simulink model "GPCA_Alarm"  (Simulink 8.5)
settings: Solver=ode45  StartTime=0.0  StopTime=10.0  RelTol=1e-3
settings Model: Creator=bourbouh  LastModifiedBy=Teme
settings DataIOCC: LimitDataPoints=off  SaveFormat=Dataset  SignalLoggingSaveFormat=Dataset
settings OptimizationCC: ExpressionDepthLimit=128
settings DebuggingCC: UnderspecifiedInitializationDetection=Simplified  MergeDetectMultiDrivingBlocksExec=error  FcnCallInpInsideContextMsg=EnableAllAsError  StateNameClashWarn=none
settings HardwareCC: ProdBitPerPointer=64  ProdLargestAtomicFloat=Float  ProdIntDivRoundTo=Zero  ProdEndianess=LittleEndian  ProdWordSize=64  ProdHWDeviceType=Intel->x86-64 (Windows64)  TargetBitPerInt=16  TargetBitPerPointer=16  TargetShiftRightIntArith=off  TargetIntDivRoundTo=Zero  TargetWordSize=8  TargetHWDeviceType=Intel->8051 Compatible  ProdEqTarget=off
settings ModelReferenceCC: PropagateSignalLabelsOutOfModel=on
settings GRTTargetCC: CombineOutputUpdateFcns=on  GRTInterface=off
settings ConfigComp: CovMetricSettings=dw  CovHtmlReporting=on  CovSaveCumulativeToWorkspaceVar=on  CovSaveSingleToWorkspaceVar=on  CovExternalEMLEnable=off

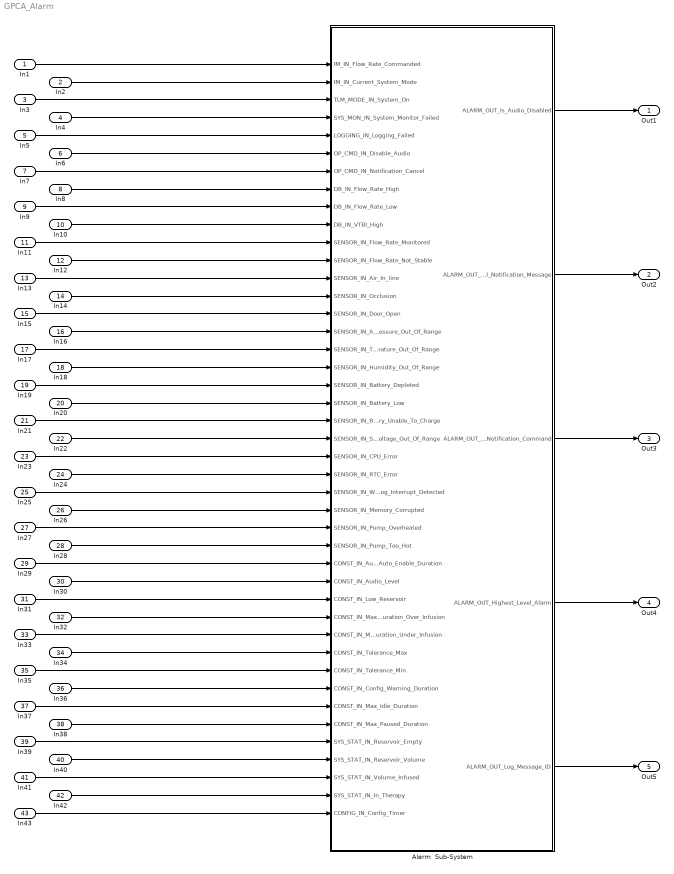
== system GPCA_Alarm ==
  In1 : Inport
  In2 : Inport  Port=2
  In3 : Inport  Port=3
  In4 : Inport  Port=4
  In5 : Inport  Port=5
  In6 : Inport  Port=6
  In7 : Inport  Port=7
  In8 : Inport  Port=8
  In9 : Inport  Port=9
  In10 : Inport  Port=10
  In11 : Inport  Port=11
  In12 : Inport  Port=12
  In13 : Inport  Port=13
  In14 : Inport  Port=14
  In15 : Inport  Port=15
  In16 : Inport  Port=16
  In17 : Inport  Port=17
  In18 : Inport  Port=18
  In19 : Inport  Port=19
  In20 : Inport  Port=20
  In21 : Inport  Port=21
  In22 : Inport  Port=22
  In23 : Inport  Port=23
  In24 : Inport  Port=24
  In25 : Inport  Port=25
  In26 : Inport  Port=26
  In27 : Inport  Port=27
  In28 : Inport  Port=28
  In29 : Inport  Port=29
  In30 : Inport  Port=30
  In31 : Inport  Port=31
  In32 : Inport  Port=32
  In33 : Inport  Port=33
  In34 : Inport  Port=34
  In35 : Inport  Port=35
  In36 : Inport  Port=36
  In37 : Inport  Port=37
  In38 : Inport  Port=38
  In39 : Inport  Port=39
  In40 : Inport  Port=40
  In41 : Inport  Port=41
  In42 : Inport  Port=42
  In43 : Inport  Port=43
  Alarm  Sub-System : Stateflow chart  TreatAsAtomicUnit=on
  Out1 : Outport
  Out2 : Outport  Port=2
  Out3 : Outport  Port=3
  Out4 : Outport  Port=4
  Out5 : Outport  Port=5
  wires:
  In1/1 -> Alarm  Sub-System/1(IM_IN_Flow_Rate_Commanded)
  In2/1 -> Alarm  Sub-System/2(IM_IN_Current_System_Mode)
  In3/1 -> Alarm  Sub-System/3(TLM_MODE_IN_System_On)
  In4/1 -> Alarm  Sub-System/4(SYS_MON_IN_System_Monitor_Failed)
  In5/1 -> Alarm  Sub-System/5(LOGGING_IN_Logging_Failed)
  In6/1 -> Alarm  Sub-System/6(OP_CMD_IN_Disable_Audio)
  In7/1 -> Alarm  Sub-System/7(OP_CMD_IN_Notification_Cancel)
  In8/1 -> Alarm  Sub-System/8(DB_IN_Flow_Rate_High)
  In9/1 -> Alarm  Sub-System/9(DB_IN_Flow_Rate_Low)
  In10/1 -> Alarm  Sub-System/10(DB_IN_VTBI_High)
  In11/1 -> Alarm  Sub-System/11(SENSOR_IN_Flow_Rate_Monitored)
  In12/1 -> Alarm  Sub-System/12(SENSOR_IN_Flow_Rate_Not_Stable)
  In13/1 -> Alarm  Sub-System/13(SENSOR_IN_Air_In_line)
  In14/1 -> Alarm  Sub-System/14(SENSOR_IN_Occlusion)
  In15/1 -> Alarm  Sub-System/15(SENSOR_IN_Door_Open)
  In16/1 -> Alarm  Sub-System/16(SENSOR_IN_Air_Pressure_Out_Of_Range)
  In17/1 -> Alarm  Sub-System/17(SENSOR_IN_Temperature_Out_Of_Range)
  In18/1 -> Alarm  Sub-System/18(SENSOR_IN_Humidity_Out_Of_Range)
  In19/1 -> Alarm  Sub-System/19(SENSOR_IN_Battery_Depleted)
  In20/1 -> Alarm  Sub-System/20(SENSOR_IN_Battery_Low)
  In21/1 -> Alarm  Sub-System/21(SENSOR_IN_Battery_Unable_To_Charge)
  In22/1 -> Alarm  Sub-System/22(SENSOR_IN_Supply_Voltage_Out_Of_Range)
  In23/1 -> Alarm  Sub-System/23(SENSOR_IN_CPU_Error)
  In24/1 -> Alarm  Sub-System/24(SENSOR_IN_RTC_Error)
  In25/1 -> Alarm  Sub-System/25(SENSOR_IN_WatchDog_Interrupt_Detected)
  In26/1 -> Alarm  Sub-System/26(SENSOR_IN_Memory_Corrupted)
  In27/1 -> Alarm  Sub-System/27(SENSOR_IN_Pump_Overheated)
  In28/1 -> Alarm  Sub-System/28(SENSOR_IN_Pump_Too_Hot)
  In29/1 -> Alarm  Sub-System/29(CONST_IN_Audio_Auto_Enable_Duration)
  In30/1 -> Alarm  Sub-System/30(CONST_IN_Audio_Level)
  In31/1 -> Alarm  Sub-System/31(CONST_IN_Low_Reservoir)
  In32/1 -> Alarm  Sub-System/32(CONST_IN_Max_Duration_Over_Infusion)
  In33/1 -> Alarm  Sub-System/33(CONST_IN_Max_Duration_Under_Infusion)
  In34/1 -> Alarm  Sub-System/34(CONST_IN_Tolerance_Max)
  In35/1 -> Alarm  Sub-System/35(CONST_IN_Tolerance_Min)
  In36/1 -> Alarm  Sub-System/36(CONST_IN_Config_Warning_Duration)
  In37/1 -> Alarm  Sub-System/37(CONST_IN_Max_Idle_Duration)
  In38/1 -> Alarm  Sub-System/38(CONST_IN_Max_Paused_Duration)
  In39/1 -> Alarm  Sub-System/39(SYS_STAT_IN_Reservoir_Empty)
  In40/1 -> Alarm  Sub-System/40(SYS_STAT_IN_Reservoir_Volume)
  In41/1 -> Alarm  Sub-System/41(SYS_STAT_IN_Volume_Infused)
  In42/1 -> Alarm  Sub-System/42(SYS_STAT_IN_In_Therapy)
  In43/1 -> Alarm  Sub-System/43(CONFIG_IN_Config_Timer)
  Alarm  Sub-System/1(ALARM_OUT_Is_Audio_Disabled) -> Out1/1
  Alarm  Sub-System/2(ALARM_OUT_Visual_Notification_Message) -> Out2/1
  Alarm  Sub-System/3(ALARM_OUT_Audio_Notification_Command) -> Out3/1
  Alarm  Sub-System/4(ALARM_OUT_Highest_Level_Alarm) -> Out4/1
  Alarm  Sub-System/5(ALARM_OUT_Log_Message_ID) -> Out5/1

== stateflow chart Alarm  Sub-System ==
  state Alarms
    state CheckAlarm [parallel]
      settings: executionOrder=1
      state CancelAlarm [parallel]
        settings: executionOrder=1
        state ON
          entry:cancelAlarm = currentAlarm;
          writeLog(3);
          during:cancelAlarm = currentAlarm;
        state OFF
        (default) -> Alarms.CheckAlarm.CancelAlarm.OFF
        Alarms.CheckAlarm.CancelAlarm.OFF -> Alarms.CheckAlarm.CancelAlarm.ON : [currentAlarm > 0 && OP_CMD_IN_Notification_Cancel]
        Alarms.CheckAlarm.CancelAlarm.ON -> Alarms.CheckAlarm.CancelAlarm.OFF
      state setHighestAlarm [function]
        (default) -> (junction 90) : {ALARM_OUT_Highest_Level_Alarm=Max_Alarm_Level;}
      state Level4 [parallel]
        settings: executionOrder=2
        state IsEmptyReservoir [parallel]
          settings: executionOrder=1
          state No
          state Yes
          (default) -> Alarms.CheckAlarm.Level4.IsEmptyReservoir.No [order 2]
          (default) -> Alarms.CheckAlarm.Level4.IsEmptyReservoir.Yes [order 1] : [SYS_STAT_IN_In_Therapy && SYS_STAT_IN_Reservoir_Empty]
          Alarms.CheckAlarm.Level4.IsEmptyReservoir.No -> Alarms.CheckAlarm.Level4.IsEmptyReservoir.Yes : [SYS_STAT_IN_In_Therapy && SYS_STAT_IN_Reservoir_Empty]
          Alarms.CheckAlarm.Level4.IsEmptyReservoir.Yes -> Alarms.CheckAlarm.Level4.IsEmptyReservoir.No [order 2] : [cancelAlarm == 1 && !SYS_STAT_IN_Reservoir_Empty]
          Alarms.CheckAlarm.Level4.IsEmptyReservoir.Yes -> Alarms.CheckAlarm.Level4.IsEmptyReservoir.Yes [order 1] : [SYS_STAT_IN_In_Therapy && SYS_STAT_IN_Reservoir_Empty]
        state IsHardwareError [parallel]
          settings: executionOrder=2
          state Yes
          state No
          (default) -> Alarms.CheckAlarm.Level4.IsHardwareError.No [order 2]
          (default) -> Alarms.CheckAlarm.Level4.IsHardwareError.Yes [order 1] : [SENSOR_IN_Battery_Depleted || SENSOR_IN_RTC_Error || SENSOR_IN_CPU_Error || SENSOR_IN_Memory_Corrupted || SENSOR_IN_Pump_Too_Hot || SENSOR_IN_WatchDog_Interrupt_Detected]
          Alarms.CheckAlarm.Level4.IsHardwareError.No -> Alarms.CheckAlarm.Level4.IsHardwareError.Yes : [SENSOR_IN_Battery_Depleted || SENSOR_IN_RTC_Error || SENSOR_IN_CPU_Error || SENSOR_IN_Memory_Corrupted || SENSOR_IN_Pump_Too_Hot || SENSOR_IN_WatchDog_Interrupt_Detected]
          Alarms.CheckAlarm.Level4.IsHardwareError.Yes -> Alarms.CheckAlarm.Level4.IsHardwareError.No : [cancelAlarm ==2 &&  ! (SENSOR_IN_Battery_Depleted || SENSOR_IN_RTC_Error || SENSOR_IN_CPU_Error || SENSOR_IN_Memory_Corrupted || SENSOR_IN_Pump_Too_Hot || SENSOR_IN_WatchDog_Interrupt_Detected)]
        state IsEnviromentalError [parallel]
          settings: executionOrder=3
          state Yes
          state No
          (default) -> Alarms.CheckAlarm.Level4.IsEnviromentalError.Yes [order 1] : [SENSOR_IN_Temperature_Out_Of_Range || SENSOR_IN_Humidity_Out_Of_Range || SENSOR_IN_Air_Pressure_Out_Of_Range]
          (default) -> Alarms.CheckAlarm.Level4.IsEnviromentalError.No [order 2]
          Alarms.CheckAlarm.Level4.IsEnviromentalError.No -> Alarms.CheckAlarm.Level4.IsEnviromentalError.Yes : [SENSOR_IN_Temperature_Out_Of_Range || SENSOR_IN_Humidity_Out_Of_Range || SENSOR_IN_Air_Pressure_Out_Of_Range]
          Alarms.CheckAlarm.Level4.IsEnviromentalError.Yes -> Alarms.CheckAlarm.Level4.IsEnviromentalError.No : [cancelAlarm == 3 && !(SENSOR_IN_Temperature_Out_Of_Range || SENSOR_IN_Humidity_Out_Of_Range || SENSOR_IN_Air_Pressure_Out_Of_Range)]
      state Level3 [parallel]
        settings: executionOrder=3
        state IsOverInfusionFlowRate [parallel]
          entry:checkOverInfusionFlowRate();
          during:checkOverInfusionFlowRate();
          exit:checkOverInfusionFlowRate();
          settings: executionOrder=1
          state Yes
            entry:overInfusion=1;
            during:overInfusion=1;
          state Check
            entry:checkOverInfusionFlowRate();
            during:checkOverInfusionFlowRate();
            exit:checkOverInfusionFlowRate();
          state Monitor
            entry:checkOverInfusionFlowRate();
            during:checkOverInfusionFlowRate();
            exit:checkOverInfusionFlowRate();
          state checkOverInfusionFlowRate [function]
            (default) -> (junction 115) : {overInfusion=0;}
            (junction 115) -> (junction 117) : [SYS_STAT_IN_In_Therapy]
            (junction 117) -> (junction 116) [order 1] : [SENSOR_IN_Flow_Rate_Monitored > DB_IN_Flow_Rate_High]{overInfusion=1;}
            (junction 117) -> (junction 118) [order 2] : [SENSOR_IN_Flow_Rate_Monitored > (IM_IN_Flow_Rate_Commanded  * ((100 + CONST_IN_Tolerance_Max)/100))]{overInfusion=1;}
            (junction 117) -> (junction 119) [order 3] : [SENSOR_IN_Flow_Rate_Monitored > (IM_IN_Flow_Rate_Commanded * ((100 + CONST_IN_Tolerance_Min) /100))]{overInfusion=2;}
          (default) -> Alarms.CheckAlarm.Level3.IsOverInfusionFlowRate.Check [order 3]
          (default) -> Alarms.CheckAlarm.Level3.IsOverInfusionFlowRate.Yes [order 1] : [overInfusion==1]
          Alarms.CheckAlarm.Level3.IsOverInfusionFlowRate.Yes -> Alarms.CheckAlarm.Level3.IsOverInfusionFlowRate.Yes [order 1] : [overInfusion==1]
          Alarms.CheckAlarm.Level3.IsOverInfusionFlowRate.Check -> Alarms.CheckAlarm.Level3.IsOverInfusionFlowRate.Yes [order 1] : [overInfusion==1]
          Alarms.CheckAlarm.Level3.IsOverInfusionFlowRate.Yes -> Alarms.CheckAlarm.Level3.IsOverInfusionFlowRate.Check [order 2] : [cancelAlarm==4]
          Alarms.CheckAlarm.Level3.IsOverInfusionFlowRate.Monitor -> Alarms.CheckAlarm.Level3.IsOverInfusionFlowRate.Yes [order 1] : [overInfusion==1 || overInfusionTimer > Step_Scaling_Factor(CONST_IN_Max_Duration_Over_Infusion, step_size)]{overInfusionTimer=0;}
          Alarms.CheckAlarm.Level3.IsOverInfusionFlowRate.Monitor -> Alarms.CheckAlarm.Level3.IsOverInfusionFlowRate.Check [order 2] : [overInfusion==0]{overInfusionTimer=0;}
          Alarms.CheckAlarm.Level3.IsOverInfusionFlowRate.Check -> Alarms.CheckAlarm.Level3.IsOverInfusionFlowRate.Monitor [order 2] : [overInfusion == 2]{overInfusionTimer=0;}
          Alarms.CheckAlarm.Level3.IsOverInfusionFlowRate.Monitor -> Alarms.CheckAlarm.Level3.IsOverInfusionFlowRate.Monitor [order 3] : [overInfusion == 2 ]{overInfusionTimer++;}
          (default) -> Alarms.CheckAlarm.Level3.IsOverInfusionFlowRate.Monitor [order 2] : [overInfusion==2]
        state IsOverInfusionVTBI [parallel]
          settings: executionOrder=2
          state Yes
          state No
          (default) -> Alarms.CheckAlarm.Level3.IsOverInfusionVTBI.Yes [order 1] : [SYS_STAT_IN_In_Therapy && SYS_STAT_IN_Volume_Infused >DB_IN_VTBI_High]
          (default) -> Alarms.CheckAlarm.Level3.IsOverInfusionVTBI.No [order 2]
          Alarms.CheckAlarm.Level3.IsOverInfusionVTBI.Yes -> Alarms.CheckAlarm.Level3.IsOverInfusionVTBI.Yes [order 1] : [SYS_STAT_IN_In_Therapy &&  SYS_STAT_IN_Volume_Infused >DB_IN_VTBI_High]
          Alarms.CheckAlarm.Level3.IsOverInfusionVTBI.No -> Alarms.CheckAlarm.Level3.IsOverInfusionVTBI.Yes : [SYS_STAT_IN_In_Therapy &&  SYS_STAT_IN_Volume_Infused >DB_IN_VTBI_High]
          Alarms.CheckAlarm.Level3.IsOverInfusionVTBI.Yes -> Alarms.CheckAlarm.Level3.IsOverInfusionVTBI.No [order 2] : [cancelAlarm==5 ]
        state IsAirInLine [parallel]
          settings: executionOrder=3
          state Yes
          state No
          (default) -> Alarms.CheckAlarm.Level3.IsAirInLine.Yes [order 1] : [SENSOR_IN_Air_In_line]
          (default) -> Alarms.CheckAlarm.Level3.IsAirInLine.No [order 2]
          Alarms.CheckAlarm.Level3.IsAirInLine.No -> Alarms.CheckAlarm.Level3.IsAirInLine.Yes : [SENSOR_IN_Air_In_line]
          Alarms.CheckAlarm.Level3.IsAirInLine.Yes -> Alarms.CheckAlarm.Level3.IsAirInLine.No : [cancelAlarm ==6 && !SENSOR_IN_Air_In_line]
        state IsOcclusion [parallel]
          settings: executionOrder=4
          state Yes
          state No
          (default) -> Alarms.CheckAlarm.Level3.IsOcclusion.Yes [order 1] : [SENSOR_IN_Occlusion]
          (default) -> Alarms.CheckAlarm.Level3.IsOcclusion.No [order 2]
          Alarms.CheckAlarm.Level3.IsOcclusion.No -> Alarms.CheckAlarm.Level3.IsOcclusion.Yes : [SENSOR_IN_Occlusion]
          Alarms.CheckAlarm.Level3.IsOcclusion.Yes -> Alarms.CheckAlarm.Level3.IsOcclusion.No : [cancelAlarm ==7 && !SENSOR_IN_Occlusion ]
        state IsDoor_Open [parallel]
          settings: executionOrder=5
          state No
          state Yes
          (default) -> Alarms.CheckAlarm.Level3.IsDoor_Open.No [order 2]
          (default) -> Alarms.CheckAlarm.Level3.IsDoor_Open.Yes [order 1] : [SENSOR_IN_Door_Open]
          Alarms.CheckAlarm.Level3.IsDoor_Open.No -> Alarms.CheckAlarm.Level3.IsDoor_Open.Yes : [SENSOR_IN_Door_Open]
          Alarms.CheckAlarm.Level3.IsDoor_Open.Yes -> Alarms.CheckAlarm.Level3.IsDoor_Open.No : [cancelAlarm ==8 && !SENSOR_IN_Door_Open]
      state Level2 [parallel]
        settings: executionOrder=4
        state IsLowReservoir [parallel]
          settings: executionOrder=1
          state No
          state Yes
          (default) -> Alarms.CheckAlarm.Level2.IsLowReservoir.No [order 2]
          (default) -> Alarms.CheckAlarm.Level2.IsLowReservoir.Yes [order 1] : [SYS_STAT_IN_In_Therapy && SYS_STAT_IN_Reservoir_Volume < CONST_IN_Low_Reservoir]
          Alarms.CheckAlarm.Level2.IsLowReservoir.No -> Alarms.CheckAlarm.Level2.IsLowReservoir.Yes : [SYS_STAT_IN_In_Therapy && SYS_STAT_IN_Reservoir_Volume < CONST_IN_Low_Reservoir]
          Alarms.CheckAlarm.Level2.IsLowReservoir.Yes -> Alarms.CheckAlarm.Level2.IsLowReservoir.No : [cancelAlarm ==9 && !(SYS_STAT_IN_Reservoir_Volume < CONST_IN_Low_Reservoir)]
      state Level1 [parallel]
        settings: executionOrder=5
        state IsUnderInfusion [parallel]
          entry: checkUnderInfusion();
          during:checkUnderInfusion();
          exit:checkUnderInfusion();
          settings: executionOrder=1
          state Yes
            entry:underInfusion=1;
            during:underInfusion=1;
          state Check
            entry: underInfusion=0;
            during:underInfusion=0;
          state Monitor
            entry:underInfusion=2;checkUnderInfusion();
            during:checkUnderInfusion();
          state checkUnderInfusion [function]
            (default) -> (junction 155) : {underInfusion=0;}
            (junction 155) -> (junction 156) : [SYS_STAT_IN_In_Therapy]
            (junction 156) -> (junction 157) [order 1] : [SENSOR_IN_Flow_Rate_Monitored < DB_IN_Flow_Rate_Low]{underInfusion=1;}
            (junction 156) -> (junction 158) [order 2] : [SENSOR_IN_Flow_Rate_Monitored < IM_IN_Flow_Rate_Commanded - (IM_IN_Flow_Rate_Commanded * (CONST_IN_Tolerance_Max/100))]{underInfusion=1;}
            (junction 156) -> (junction 159) [order 3] : [SENSOR_IN_Flow_Rate_Monitored < IM_IN_Flow_Rate_Commanded - (IM_IN_Flow_Rate_Commanded * (CONST_IN_Tolerance_Min/100))]{underInfusion=2;}
          (default) -> Alarms.CheckAlarm.Level1.IsUnderInfusion.Yes [order 1] : [underInfusion==1]
          (default) -> Alarms.CheckAlarm.Level1.IsUnderInfusion.Check [order 3]
          Alarms.CheckAlarm.Level1.IsUnderInfusion.Check -> Alarms.CheckAlarm.Level1.IsUnderInfusion.Yes [order 1] : [underInfusion==1]
          Alarms.CheckAlarm.Level1.IsUnderInfusion.Yes -> Alarms.CheckAlarm.Level1.IsUnderInfusion.Check : [cancelAlarm==10]
          Alarms.CheckAlarm.Level1.IsUnderInfusion.Monitor -> Alarms.CheckAlarm.Level1.IsUnderInfusion.Yes [order 1] : [underInfusion==1 ||underInfusionTimer > Step_Scaling_Factor(CONST_IN_Max_Duration_Under_Infusion, step_size)] {underInfusionTimer=0;}
          Alarms.CheckAlarm.Level1.IsUnderInfusion.Monitor -> Alarms.CheckAlarm.Level1.IsUnderInfusion.Check [order 3] : [underInfusion==0]{underInfusionTimer=0;}
          Alarms.CheckAlarm.Level1.IsUnderInfusion.Check -> Alarms.CheckAlarm.Level1.IsUnderInfusion.Monitor [order 2] : [underInfusion==2]{underInfusionTimer=0;}
          (default) -> Alarms.CheckAlarm.Level1.IsUnderInfusion.Monitor [order 2] : [underInfusion==2]
          Alarms.CheckAlarm.Level1.IsUnderInfusion.Monitor -> Alarms.CheckAlarm.Level1.IsUnderInfusion.Monitor [order 2] : [underInfusion==2]{underInfusionTimer++;}
        state IsFlowRateNotStable [parallel]
          settings: executionOrder=2
          state Yes
          state No
          (default) -> Alarms.CheckAlarm.Level1.IsFlowRateNotStable.Yes [order 1] : [SYS_STAT_IN_In_Therapy && SENSOR_IN_Flow_Rate_Not_Stable]
          (default) -> Alarms.CheckAlarm.Level1.IsFlowRateNotStable.No [order 2]
          Alarms.CheckAlarm.Level1.IsFlowRateNotStable.No -> Alarms.CheckAlarm.Level1.IsFlowRateNotStable.Yes : [SYS_STAT_IN_In_Therapy && SENSOR_IN_Flow_Rate_Not_Stable]
          Alarms.CheckAlarm.Level1.IsFlowRateNotStable.Yes -> Alarms.CheckAlarm.Level1.IsFlowRateNotStable.No : [cancelAlarm==11 && !SENSOR_IN_Flow_Rate_Not_Stable]
        state IsPausedTimeExceeded [parallel]
          settings: executionOrder=4
          state counting
            entry: pausedtimer++;
            during: pausedtimer++;
            exit: pausedtimer++;
          state No
            entry:pausedtimer=0;
            during:pausedtimer=0;
            exit:pausedtimer=0;
          state Yes
          (default) -> Alarms.CheckAlarm.Level1.IsPausedTimeExceeded.counting [order 2] : [IM_IN_Current_System_Mode == 6 || IM_IN_Current_System_Mode == 7 ||  IM_IN_Current_System_Mode == 8 ]{pausedtimer=0;}
          (default) -> Alarms.CheckAlarm.Level1.IsPausedTimeExceeded.No [order 3]
          Alarms.CheckAlarm.Level1.IsPausedTimeExceeded.No -> Alarms.CheckAlarm.Level1.IsPausedTimeExceeded.counting [order 2] : [IM_IN_Current_System_Mode == 6 || IM_IN_Current_System_Mode == 7 ||  IM_IN_Current_System_Mode == 8 ]{pausedtimer=0;}
          Alarms.CheckAlarm.Level1.IsPausedTimeExceeded.Yes -> Alarms.CheckAlarm.Level1.IsPausedTimeExceeded.No : [cancelAlarm==13]
          Alarms.CheckAlarm.Level1.IsPausedTimeExceeded.No -> Alarms.CheckAlarm.Level1.IsPausedTimeExceeded.Yes [order 1] : [(IM_IN_Current_System_Mode == 6 || IM_IN_Current_System_Mode == 7 ||  IM_IN_Current_System_Mode == 8 ) &&  Step_Scaling_Factor(CONST_IN_Max_Paused_Duration,step_size) == 1]
          Alarms.CheckAlarm.Level1.IsPausedTimeExceeded.counting -> Alarms.CheckAlarm.Level1.IsPausedTimeExceeded.Yes : [ pausedtimer >= Step_Scaling_Factor(CONST_IN_Max_Paused_Duration,step_size)]
          (default) -> Alarms.CheckAlarm.Level1.IsPausedTimeExceeded.Yes [order 1] : [(IM_IN_Current_System_Mode == 6 || IM_IN_Current_System_Mode == 7 ||  IM_IN_Current_System_Mode == 8 ) &&  Step_Scaling_Factor(CONST_IN_Max_Paused_Duration,step_size) == 1]
        state IsIdleTimeExceeded [parallel]
          settings: executionOrder=3
          state counting
            entry: idletimer++;
            during: idletimer++;
            exit: idletimer++;
          state No
            entry:idletimer=0;
            during:idletimer=0;
            exit:idletimer=0;
          state Yes
          (default) -> Alarms.CheckAlarm.Level1.IsIdleTimeExceeded.counting [order 2] : [IM_IN_Current_System_Mode == 1]{idletimer=0;}
          (default) -> Alarms.CheckAlarm.Level1.IsIdleTimeExceeded.No [order 3]
          Alarms.CheckAlarm.Level1.IsIdleTimeExceeded.No -> Alarms.CheckAlarm.Level1.IsIdleTimeExceeded.counting [order 2] : [IM_IN_Current_System_Mode == 1]{idletimer=0;}
          Alarms.CheckAlarm.Level1.IsIdleTimeExceeded.No -> Alarms.CheckAlarm.Level1.IsIdleTimeExceeded.Yes [order 1] : [IM_IN_Current_System_Mode == 1 &&  Step_Scaling_Factor(CONST_IN_Max_Idle_Duration,step_size) == 1]
          Alarms.CheckAlarm.Level1.IsIdleTimeExceeded.Yes -> Alarms.CheckAlarm.Level1.IsIdleTimeExceeded.No : [cancelAlarm==12]
          Alarms.CheckAlarm.Level1.IsIdleTimeExceeded.counting -> Alarms.CheckAlarm.Level1.IsIdleTimeExceeded.Yes : [ idletimer >= Step_Scaling_Factor(CONST_IN_Max_Idle_Duration,step_size)]
          (default) -> Alarms.CheckAlarm.Level1.IsIdleTimeExceeded.Yes [order 1] : [IM_IN_Current_System_Mode == 1 &&  Step_Scaling_Factor(CONST_IN_Max_Idle_Duration,step_size) == 1]
        state IsConfigTimeWarning [parallel]
          settings: executionOrder=5
          state No
          state Yes
          (default) -> Alarms.CheckAlarm.Level1.IsConfigTimeWarning.No [order 2]
          (default) -> Alarms.CheckAlarm.Level1.IsConfigTimeWarning.Yes [order 1] : [CONFIG_IN_Config_Timer > Step_Scaling_Factor(CONST_IN_Config_Warning_Duration, step_size)]
          Alarms.CheckAlarm.Level1.IsConfigTimeWarning.No -> Alarms.CheckAlarm.Level1.IsConfigTimeWarning.Yes : [CONFIG_IN_Config_Timer > Step_Scaling_Factor(CONST_IN_Config_Warning_Duration, step_size)]
          Alarms.CheckAlarm.Level1.IsConfigTimeWarning.Yes -> Alarms.CheckAlarm.Level1.IsConfigTimeWarning.No : [cancelAlarm==14 && !(CONFIG_IN_Config_Timer > Step_Scaling_Factor(CONST_IN_Config_Warning_Duration, step_size))]
        state IsBatteryError [parallel]
          settings: executionOrder=6
          state Yes
          state No
          (default) -> Alarms.CheckAlarm.Level1.IsBatteryError.Yes [order 1] : [SENSOR_IN_Battery_Low || SENSOR_IN_Battery_Unable_To_Charge || SENSOR_IN_Supply_Voltage_Out_Of_Range]
          (default) -> Alarms.CheckAlarm.Level1.IsBatteryError.No [order 2]
          Alarms.CheckAlarm.Level1.IsBatteryError.No -> Alarms.CheckAlarm.Level1.IsBatteryError.Yes : [SENSOR_IN_Battery_Low || SENSOR_IN_Battery_Unable_To_Charge || SENSOR_IN_Supply_Voltage_Out_Of_Range]
          Alarms.CheckAlarm.Level1.IsBatteryError.Yes -> Alarms.CheckAlarm.Level1.IsBatteryError.No : [cancelAlarm==15 &&  !(SENSOR_IN_Battery_Low || SENSOR_IN_Battery_Unable_To_Charge || SENSOR_IN_Supply_Voltage_Out_Of_Range)]
        state IsPumpHot [parallel]
          settings: executionOrder=7
          state Yes
          state No
          (default) -> Alarms.CheckAlarm.Level1.IsPumpHot.Yes [order 1] : [SENSOR_IN_Pump_Overheated]
          (default) -> Alarms.CheckAlarm.Level1.IsPumpHot.No [order 2]
          Alarms.CheckAlarm.Level1.IsPumpHot.No -> Alarms.CheckAlarm.Level1.IsPumpHot.Yes : [SENSOR_IN_Pump_Overheated]
          Alarms.CheckAlarm.Level1.IsPumpHot.Yes -> Alarms.CheckAlarm.Level1.IsPumpHot.No : [cancelAlarm==16 && !SENSOR_IN_Pump_Overheated]
        state IsLoggingFailed [parallel]
          settings: executionOrder=8
          state Yes
          state No
          (default) -> Alarms.CheckAlarm.Level1.IsLoggingFailed.Yes [order 1] : [LOGGING_IN_Logging_Failed ]
          (default) -> Alarms.CheckAlarm.Level1.IsLoggingFailed.No [order 2]
          Alarms.CheckAlarm.Level1.IsLoggingFailed.No -> Alarms.CheckAlarm.Level1.IsLoggingFailed.Yes : [LOGGING_IN_Logging_Failed ]
          Alarms.CheckAlarm.Level1.IsLoggingFailed.Yes -> Alarms.CheckAlarm.Level1.IsLoggingFailed.No : [cancelAlarm==17 && !LOGGING_IN_Logging_Failed ]
        state IsSystemMonitorFailed [parallel]
          settings: executionOrder=9
          state Yes
          state No
          (default) -> Alarms.CheckAlarm.Level1.IsSystemMonitorFailed.Yes [order 1] : [SYS_MON_IN_System_Monitor_Failed]
          (default) -> Alarms.CheckAlarm.Level1.IsSystemMonitorFailed.No [order 2]
          Alarms.CheckAlarm.Level1.IsSystemMonitorFailed.No -> Alarms.CheckAlarm.Level1.IsSystemMonitorFailed.Yes : [SYS_MON_IN_System_Monitor_Failed]
          Alarms.CheckAlarm.Level1.IsSystemMonitorFailed.Yes -> Alarms.CheckAlarm.Level1.IsSystemMonitorFailed.No : [cancelAlarm==18 && !SYS_MON_IN_System_Monitor_Failed]
      state SetAlarmStatus [parallel]
        entry:setHighestAlarm();
        during:setHighestAlarm();
        exit:setHighestAlarm();
        cancelAlarm=0;
        settings: executionOrder=6
    state Notification [parallel]
      settings: executionOrder=2
      state Visual [parallel]
        settings: executionOrder=1
        state OFF
          entry:ALARM_OUT_Visual_Notification_Message = 0;
          previousAlarm=0;
        state AlarmDisplay
          entry:ALARM_OUT_Visual_Notification_Message = currentAlarm;
          during:ALARM_OUT_Visual_Notification_Message = currentAlarm;
          exit:ALARM_OUT_Visual_Notification_Message = currentAlarm;
        (default) -> Alarms.Notification.Visual.OFF [order 2]
        (default) -> AlarmDisplay [order 1] : [currentAlarm > 0]
        Alarms.Notification.Visual.OFF -> AlarmDisplay : [currentAlarm > 0]
        AlarmDisplay -> Alarms.Notification.Visual.OFF [order 1] : [currentAlarm == 0]
        AlarmDisplay -> AlarmDisplay [order 2] : [currentAlarm > 0]
      state Audio [parallel]
        entry: ALARM_OUT_Is_Audio_Disabled=OP_CMD_IN_Disable_Audio;
        during: ALARM_OUT_Is_Audio_Disabled=OP_CMD_IN_Disable_Audio;
        exit: ALARM_OUT_Is_Audio_Disabled=OP_CMD_IN_Disable_Audio;
        settings: executionOrder=2
        state ON
          entry: ALARM_OUT_Audio_Notification_Command=CONST_IN_Audio_Level;
          during: ALARM_OUT_Audio_Notification_Command=CONST_IN_Audio_Level;
          exit: ALARM_OUT_Audio_Notification_Command=CONST_IN_Audio_Level;
        state OFF
          entry: ALARM_OUT_Audio_Notification_Command=0;
          during: ALARM_OUT_Audio_Notification_Command=0;
          exit: ALARM_OUT_Audio_Notification_Command=0;
        state Silenced
          entry: audioTimer = 0;ALARM_OUT_Audio_Notification_Command=0;audioTimer++;
          exit: ALARM_OUT_Audio_Notification_Command=0;
          during: audioTimer++;ALARM_OUT_Audio_Notification_Command=0;
        state Disabled
          entry: ALARM_OUT_Audio_Notification_Command=0;
          during: ALARM_OUT_Audio_Notification_Command=0;
          exit: ALARM_OUT_Audio_Notification_Command=0;
        (default) -> Alarms.Notification.Audio.OFF [order 4]
        Alarms.Notification.Audio.ON -> Alarms.Notification.Audio.ON [order 3] : [ALARM_OUT_Highest_Level_Alarm > 2 && OP_CMD_IN_Disable_Audio == 0]
        (default) -> Alarms.Notification.Audio.ON [order 3] : [ALARM_OUT_Highest_Level_Alarm > 2 && OP_CMD_IN_Disable_Audio == 0]
        Alarms.Notification.Audio.OFF -> Alarms.Notification.Audio.ON [order 3] : [ALARM_OUT_Highest_Level_Alarm > 2 && OP_CMD_IN_Disable_Audio == 0]
        Alarms.Notification.Audio.ON -> Alarms.Notification.Audio.OFF [order 4]
        (junction 209) -> Alarms.Notification.Audio.OFF
        Alarms.Notification.Audio.OFF -> (junction 208) [order 2]
        Alarms.Notification.Audio.OFF -> Disabled [order 1] : [OP_CMD_IN_Disable_Audio == 1]
        Alarms.Notification.Audio.ON -> Disabled [order 1] : [OP_CMD_IN_Disable_Audio == 1]
        Alarms.Notification.Audio.ON -> (junction 208) [order 2]
        (junction 210) -> Alarms.Notification.Audio.ON : [ALARM_OUT_Highest_Level_Alarm > 2 && OP_CMD_IN_Disable_Audio == 0]
        (junction 208) -> Silenced : [OP_CMD_IN_Disable_Audio == 2]
        Silenced -> (junction 209) [order 3] : [(audioTimer > Step_Scaling_Factor(CONST_IN_Audio_Auto_Enable_Duration,step_size)) || OP_CMD_IN_Disable_Audio == 0]
        Silenced -> (junction 210) [order 2]
        Disabled -> (junction 209) [order 3] : [OP_CMD_IN_Disable_Audio == 0]
        Disabled -> (junction 210) [order 2]
        Silenced -> Disabled [order 1] : [OP_CMD_IN_Disable_Audio == 1]
        (default) -> Silenced [order 2] : [OP_CMD_IN_Disable_Audio ==2]
        Disabled -> Silenced [order 1] : [OP_CMD_IN_Disable_Audio == 2]
        (default) -> Disabled [order 1] : [OP_CMD_IN_Disable_Audio ==1]
  note: step scaling factor returns the scaled time depending upon the step size.
      | If counter has to timeout after 100 seconds and if the step size is 0.1 second
      | the new timeout value = 100/0.1 = 1000 steps.
      | default will be one step = 1 second.
  state NOT_ON
  state writeLog(logEvent) [function]
    (default) -> (junction 232) : {ALARM_OUT_Log_Message_ID=logEvent;}
  state returnVal = Step_Scaling_Factor(inputVal,step_size) [function]
    (default) -> (junction 237) : {returnVal=uint8(double(inputVal)/step_size);}
  (default) -> Alarms [order 1] : [TLM_MODE_IN_System_On]
  (default) -> NOT_ON [order 2]
  NOT_ON -> Alarms : [TLM_MODE_IN_System_On]
  Alarms -> NOT_ON : [!TLM_MODE_IN_System_On]
  data: logEvent function_input uint8; inputVal function_input uint8; returnVal function_output uint8; step_size function_input double; IM_IN_Flow_Rate_Commanded input uint8; IM_IN_Current_System_Mode input uint8; TLM_MODE_IN_System_On input boolean; SYS_MON_IN_System_Monitor_Failed input boolean; LOGGING_IN_Logging_Failed input boolean; OP_CMD_IN_Disable_Audio input uint8; OP_CMD_IN_Notification_Cancel input boolean; DB_IN_Flow_Rate_High input uint8; DB_IN_Flow_Rate_Low input uint8; DB_IN_VTBI_High input uint8; SENSOR_IN_Flow_Rate_Monitored input uint8; SENSOR_IN_Flow_Rate_Not_Stable input boolean; SENSOR_IN_Air_In_line input boolean; SENSOR_IN_Occlusion input boolean; SENSOR_IN_Door_Open input boolean; ALARM_OUT_Is_Audio_Disabled output uint8; ALARM_OUT_Visual_Notification_Message output uint8; ALARM_OUT_Audio_Notification_Command output uint8; overInfusion local uint8; overInfusionTimer local uint8; underInfusion local uint8; underInfusionTimer local uint8; ALARM_OUT_Highest_Level_Alarm output uint8; ALARM_OUT_Log_Message_ID output uint8; currentAlarm local uint8; previousAlarm local uint8; SENSOR_IN_Air_Pressure_Out_Of_Range input boolean; SENSOR_IN_Temperature_Out_Of_Range input boolean; SENSOR_IN_Humidity_Out_Of_Range input boolean; SENSOR_IN_Battery_Depleted input boolean; SENSOR_IN_Battery_Low input boolean; SENSOR_IN_Battery_Unable_To_Charge input boolean; SENSOR_IN_Supply_Voltage_Out_Of_Range input boolean; SENSOR_IN_CPU_Error input boolean; SENSOR_IN_RTC_Error input boolean; SENSOR_IN_WatchDog_Interrupt_Detected input boolean; SENSOR_IN_Memory_Corrupted input boolean; SENSOR_IN_Pump_Overheated input boolean; SENSOR_IN_Pump_Too_Hot input boolean; CONST_IN_Audio_Auto_Enable_Duration input uint8; CONST_IN_Audio_Level input uint8; CONST_IN_Low_Reservoir input uint8; CONST_IN_Max_Duration_Over_Infusion input uint8; CONST_IN_Max_Duration_Under_Infusion input uint8; CONST_IN_Tolerance_Max input uint8; CONST_IN_Tolerance_Min input uint8; CONST_IN_Config_Warning_Duration input uint8; CONST_IN_Max_Idle_Duration input uint8; CONST_IN_Max_Paused_Duration input uint8; audioTimer local uint8; cancelAlarm local uint8; SYS_STAT_IN_Reservoir_Empty input boolean; SYS_STAT_IN_Reservoir_Volume input uint8; SYS_STAT_IN_Volume_Infused input uint8; SYS_STAT_IN_In_Therapy input boolean; Max_Alarm_Level local uint8; CONFIG_IN_Config_Timer input uint8; idletimer local uint8; pausedtimer local uint8; step_size parameter double
